simulink library "gnss_sdr_tcp_connector_tracking_lib"  (Simulink 7.6)
settings: Solver=VariableStepDiscrete  StartTime=0.0  StopTime=10.0  RelTol=1e-3
undefined symbols (not defined in the file or in its folder): B_DLL, B_PLL, f0, magnitude, SFunSlope, T, Tc, Ti
libraries: simulink x518, instrumentlib x2, dspindex x1
(part 1 of 4)
settings Model: Creator=David Pubill  LastModifiedBy=gnss

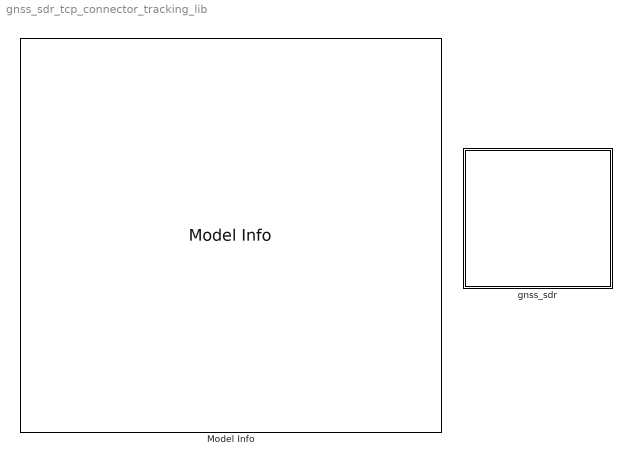
== system gnss_sdr_tcp_connector_tracking_lib ==
  Model Info : simulink/Model-Wide Utilities/Model Info  SystemSampleTime=-1  InitialBlockCM=None  BlockCM=None  Frame=on  DisplayStringWithTags=|  HorizontalTextAlignment=Left  LeftAlignmentValue=0.02  SourceBlockDiagram=gnss_sdr_tcp_connector_tracking_lib  TagMaxNumber=20
      | /*! 
      |   * \file gnss_sdr_tcp_connector_tracking_lib.mdl
      |   * \brief  gnss_sdr_tcp_connector_tracking Simulink library model. For 
      |   * further information, please check  the README_gnss_sdr_tcp_connector_tracking.txt
      |   * file or the README_gnss_sdr_tcp_connector_parallel_tracking.txt
      |   * file for parallel computing execution.
      |   *
      |   * \author David Pubill, 2012. dpubill(at)cttc.es
      |   * -------------------------------------------------------------------------
      |   *
      |   * Copyright (C) 2010-2012  (see AUTHORS file for a list of contributors)
      |   *
      |   * GNSS-SDR is a software defined Global Navigation
      |   *          Satellite Systems receiver
      |   *
      |   * This file is part of GNSS-SDR.
      |   *
      |   * GNSS-SDR is free software: you can redistribute it and/or modify
      |   * it under the terms of the GNU General Public License as published by
      |   * the Free Software Foundation, either version 3 of the License, or
      |   * at your option) any later version.
      |   *
      |   * GNSS-SDR is distributed in the hope that it will be useful,
      |   * but WITHOUT ANY WARRANTY; without even the implied warranty of
      |   * MERCHANTABILITY or FITNESS FOR A PARTICULAR PURPOSE.  See the
      |   * GNU General Public License for more details.
      |   *
      |   * You should have received a copy of the GNU General Public License
      |   * along with GNSS-SDR. If not, see <http://www.gnu.org/licenses/>.
      |   *
      |   * -------------------------------------------------------------------------
      |   */
  gnss_sdr : Subsystem

== system gnss_sdr_tcp_connector_tracking_lib/gnss_sdr ==
  gnss_sdr_tcp_connector_tracking : Subsystem  AncestorBlock=simulink/User-Defined Functions/gnss_sdr/gnss_sdr_tcp_connector_tracking
  gnss_sdr_tcp_connector_tracking_rx : Subsystem
  gnss_sdr_tcp_connector_tracking_tx : Subsystem  AncestorBlock=simulink/User-Defined Functions/gnss_sdr/gnss_sdr_tcp_connector_tracking_tx

== system gnss_sdr_tcp_connector_tracking_lib/gnss_sdr/gnss_sdr_tcp_connector_tracking ==
  control_id : Inport
  d_E_I : Inport  Port=2
  d_E_Q : Inport  Port=3
  d_L_I : Inport  Port=4
  d_L_Q : Inport  Port=5
  d_P_I : Inport  Port=6
  d_P_Q : Inport  Port=7
  d_acq_carrier_doppler_[Hz] : Inport  Port=8
  enable_tracking : Inport  Port=9
  Abs : Abs
  Abs1 : Abs
  Abs2 : Abs
  Carrier Tracking  (PLL) : Subsystem
  Code Tracking (DLL) : Subsystem
  Data Type  Conversion1 : DataTypeConversion  OutDataTypeStr=single  SaturateOnIntegerOverflow=on  RndMeth=Zero
  Data Type  Conversion2 : DataTypeConversion  OutDataTypeStr=double  SaturateOnIntegerOverflow=on  RndMeth=Zero
  Data Type  Conversion3 : DataTypeConversion  OutDataTypeStr=single  SaturateOnIntegerOverflow=on  RndMeth=Zero
  Data Type  Conversion4 : DataTypeConversion  OutDataTypeStr=single  SaturateOnIntegerOverflow=on  RndMeth=Zero
  Data Type  Conversion5 : DataTypeConversion  OutDataTypeStr=double  SaturateOnIntegerOverflow=on  RndMeth=Zero
  Data Type  Conversion6 : DataTypeConversion  OutDataTypeStr=double  SaturateOnIntegerOverflow=on  RndMeth=Zero
  Mux : Mux  Inputs=3
  Real-Imag to Complex : RealImagToComplex
  Real-Imag to Complex1 : RealImagToComplex
  Real-Imag to Complex2 : RealImagToComplex
  "[rad/s] to [Hz]" : Gain  Gain=1/(2*pi)
  control_id_ : Outport
  code_error_[s] : Outport  Port=2
  carrier_error : Outport  Port=3
  carrier_doppler_[Hz] : Outport  Port=4
  EPL Scope : Outport  Port=5
  wires:
  Carrier Tracking  (PLL)/2(carrier_doppler) -> Code Tracking (DLL)/4(carrier_aid), "[rad/s] to [Hz]"/1
  Code Tracking (DLL)/1(code_error [s]) -> Data Type  Conversion1/1
  Real-Imag to Complex/1 -> Data Type  Conversion2/1
  Carrier Tracking  (PLL)/1(carrier_error) -> Data Type  Conversion4/1
  Real-Imag to Complex1/1 -> Data Type  Conversion5/1
  Real-Imag to Complex2/1 -> Data Type  Conversion6/1
  d_E_I/1 -> Real-Imag to Complex/1
  d_E_Q/1 -> Real-Imag to Complex/2
  Data Type  Conversion1/1 -> code_error_[s]/1
  Data Type  Conversion4/1 -> carrier_error/1
  control_id/1 -> control_id_/1
  d_L_I/1 -> Real-Imag to Complex1/1
  d_L_Q/1 -> Real-Imag to Complex1/2
  d_P_I/1 -> Real-Imag to Complex2/1
  d_P_Q/1 -> Real-Imag to Complex2/2
  Data Type  Conversion2/1 -> Code Tracking (DLL)/1(E), Abs2/1
  Data Type  Conversion5/1 -> Code Tracking (DLL)/3(L), Abs/1
  Data Type  Conversion6/1 -> Carrier Tracking  (PLL)/1(P), Code Tracking (DLL)/2(P), Abs1/1
  d_acq_carrier_doppler_[Hz]/1 -> Carrier Tracking  (PLL)/2(d_acq_carrier_doppler_[Hz])
  "[rad/s] to [Hz]"/1 -> Data Type  Conversion3/1
  Data Type  Conversion3/1 -> carrier_doppler_[Hz]/1
  enable_tracking/1 -> Carrier Tracking  (PLL)/3(enable_tracking)
  Abs/1 -> Mux/3
  Abs1/1 -> Mux/2
  Abs2/1 -> Mux/1
  Mux/1 -> EPL Scope/1

== system gnss_sdr_tcp_connector_tracking_lib/gnss_sdr/gnss_sdr_tcp_connector_tracking_rx ==
  Multiport Selector : dspindex/Multiport Selector  rowsOrCols=Rows  idxCellArray={1,2,3,4,5,6,7,8,9,10,11,12,13,14,15,16,17,18,19,20,21,22,23,24,25,26,27,28,29,30,31,32,33,34,35,36}  idxErrMode=Clip Index
  RX : instrumentlib/TCP//IP Receive  DialogController=instrumentcreatedialog  DialogControllerArgs=DataTag4  Host=84.88.61.86  Port=2070  DataSize=36  EnableBlockingMode=on  Timeout=5  SampleTime=-1  DataType=uint8  ByteOrder=BigEndian
  Subsystem : Subsystem
  Subsystem1 : Subsystem
  Subsystem2 : Subsystem
  Subsystem3 : Subsystem
  Subsystem4 : Subsystem
  Subsystem5 : Subsystem
  Subsystem6 : Subsystem
  Subsystem7 : Subsystem
  Subsystem8 : Subsystem
  control_id : Outport
  d_E_I : Outport  Port=2
  d_E_Q : Outport  Port=3
  d_L_I : Outport  Port=4
  d_L_Q : Outport  Port=5
  d_P_I : Outport  Port=6
  d_P_Q : Outport  Port=7
  d_acq_carrier_doppler_hz : Outport  Port=8
  enable_tracking : Outport  Port=9
  wires:
  RX/1 -> Multiport Selector/1
  Multiport Selector/1 -> Subsystem8/1(In1)
  Multiport Selector/2 -> Subsystem8/2(In2)
  Multiport Selector/3 -> Subsystem8/3(In3)
  Multiport Selector/4 -> Subsystem8/4(In4)
  Multiport Selector/5 -> Subsystem/1(In1)
  Multiport Selector/6 -> Subsystem/2(In2)
  Multiport Selector/7 -> Subsystem/3(In3)
  Multiport Selector/8 -> Subsystem/4(In4)
  Multiport Selector/9 -> Subsystem1/1(In1)
  Multiport Selector/10 -> Subsystem1/2(In2)
  Multiport Selector/11 -> Subsystem1/3(In3)
  Multiport Selector/12 -> Subsystem1/4(In4)
  Multiport Selector/13 -> Subsystem2/1(In1)
  Multiport Selector/14 -> Subsystem2/2(In2)
  Multiport Selector/15 -> Subsystem2/3(In3)
  Multiport Selector/16 -> Subsystem2/4(In4)
  Multiport Selector/17 -> Subsystem3/1(In1)
  Multiport Selector/18 -> Subsystem3/2(In2)
  Multiport Selector/19 -> Subsystem3/3(In3)
  Multiport Selector/20 -> Subsystem3/4(In4)
  Multiport Selector/21 -> Subsystem4/1(In1)
  Multiport Selector/22 -> Subsystem4/2(In2)
  Multiport Selector/23 -> Subsystem4/3(In3)
  Multiport Selector/24 -> Subsystem4/4(In4)
  Multiport Selector/25 -> Subsystem5/1(In1)
  Multiport Selector/26 -> Subsystem5/2(In2)
  Multiport Selector/27 -> Subsystem5/3(In3)
  Multiport Selector/28 -> Subsystem5/4(In4)
  Subsystem4/1(d_P_I) -> d_P_I/1
  Subsystem3/1(d_L_Q) -> d_L_Q/1
  Subsystem2/1(d_L_I) -> d_L_I/1
  Subsystem1/1(d_E_Q) -> d_E_Q/1
  Subsystem/1(d_E_I) -> d_E_I/1
  Subsystem8/1(control_id) -> control_id/1
  Subsystem5/1(d_P_Q) -> d_P_Q/1
  Multiport Selector/29 -> Subsystem6/1(In1)
  Multiport Selector/30 -> Subsystem6/2(In2)
  Multiport Selector/31 -> Subsystem6/3(In3)
  Multiport Selector/32 -> Subsystem6/4(In4)
  Subsystem6/1(d_acq_carrier_doppler_hz) -> d_acq_carrier_doppler_hz/1
  Subsystem7/1(enable_tracking) -> enable_tracking/1
  Multiport Selector/33 -> Subsystem7/1(In1)
  Multiport Selector/34 -> Subsystem7/2(In2)
  Multiport Selector/35 -> Subsystem7/3(In3)
  Multiport Selector/36 -> Subsystem7/4(In4)

== system gnss_sdr_tcp_connector_tracking_lib/gnss_sdr/gnss_sdr_tcp_connector_tracking_tx ==
  control_id : Inport
  code_error : Inport  Port=2
  carr_error : Inport  Port=3
  carrier_doppler_hz : Inport  Port=4
  Display : Display
  TX : instrumentlib/TCP//IP Send  DialogController=instrumentcreatedialog  DialogControllerArgs=DataTag5  Host=84.88.61.86  Port=2070  EnableBlockingMode=on  Timeout=10  ByteOrder=LittleEndian
  Vector Concatenate1 : Concatenate  NumInputs=4  Mode=Vector
  wires:
  carr_error/1 -> Vector Concatenate1/3
  code_error/1 -> Vector Concatenate1/2
  control_id/1 -> Vector Concatenate1/1
  Vector Concatenate1/1 -> TX/1, Display/1
  carrier_doppler_hz/1 -> Vector Concatenate1/4

== system gnss_sdr_tcp_connector_tracking_lib/gnss_sdr/gnss_sdr_tcp_connector_tracking/Carrier Tracking  (PLL) ==
  P : Inport
  d_acq_carrier_doppler_[Hz] : Inport  Port=2
  enable_tracking : Inport  Port=3
  Data Type  Conversion2 : DataTypeConversion  OutDataTypeStr=double  SaturateOnIntegerOverflow=on  RndMeth=Zero
  Delay : simulink/Discrete/Integer Delay  NumDelays=1  InputProcessing=Inherited  vinit=0.0  samptime=Ti
  Error Accumulator : Subsystem
  First-Order Low-Pass Filter : Subsystem
  PLL Costas loop two  quadrant arctan discriminator : Subsystem  AncestorBlock=|
      | gnss_sdr_tcp_connector_tracking_lib/gnss_sdr/gnss_sdr_tcp_connector_tracking/Carrier Tracking 
      | (PLL)/atan2(Q,I)1/PLL Costas loop two quadrant arctan discriminator
  Sum : Sum  Inputs=|++
  Sum2 : Sum  Inputs=++|
  "[Hz] to [rad/Ti]" : Gain  Gain=2*pi*Ti  SaturateOnIntegerOverflow=on  OutDataTypeStr=Inherit: Same as input  ParamDataTypeStr=Inherit: Same as input
  "[rad/Ti] to [rad/s]" : Gain  Gain=1/Ti
  carrier_error : Outport
  carrier_doppler : Outport  Port=2
  wires:
  Sum/1 -> Error Accumulator/1(e)
  Error Accumulator/1(sum(e)) -> carrier_error/1
  P/1 -> PLL Costas loop two  quadrant arctan discriminator/1(In)
  "[rad/Ti] to [rad/s]"/1 -> carrier_doppler/1
  Delay/1 -> Sum/2
  Sum2/1 -> "[rad/Ti] to [rad/s]"/1
  d_acq_carrier_doppler_[Hz]/1 -> Data Type  Conversion2/1
  Data Type  Conversion2/1 -> "[Hz] to [rad/Ti]"/1
  enable_tracking/1 -> Error Accumulator/2(enable_tracking)
  "[Hz] to [rad/Ti]"/1 -> Delay/1, Sum2/2
  First-Order Low-Pass Filter/1(Out) -> Sum/1, Sum2/1
  PLL Costas loop two  quadrant arctan discriminator/1(Out) -> First-Order Low-Pass Filter/1(In)

== system gnss_sdr_tcp_connector_tracking_lib/gnss_sdr/gnss_sdr_tcp_connector_tracking/Code Tracking (DLL) ==
  E : Inport
  P : Inport  Port=2
  L : Inport  Port=3
  carrier_aid : Inport  Port=4
  Delay : simulink/Discrete/Integer Delay  NumDelays=1  InputProcessing=Inherited  vinit=0.0  samptime=Ti
  Early-Late Power : Subsystem
  Gain : Gain  Gain=-1
  Normalization : Subsystem
  Sum : Sum  Inputs=|++
  Terminator : Terminator
  Zero Order Low-Pass Filter : Subsystem
  "[chip] to [s]" : Gain  Gain=Tc  SaturateOnIntegerOverflow=on  OutDataTypeStr=Inherit: Same as input  ParamDataTypeStr=Inherit: Same as input
  "[rad/s] to [s/Ti]" : Gain  Gain=-Ti/(2*pi*f0)
  code_error [s] : Outport
  wires:
  Gain/1 -> Zero Order Low-Pass Filter/1(in)
  L/1 -> Normalization/3(L)
  P/1 -> Normalization/2(P)
  E/1 -> Normalization/1(E)
  "[chip] to [s]"/1 -> Gain/1
  Early-Late Power/1(Tau) -> "[chip] to [s]"/1
  "[rad/s] to [s/Ti]"/1 -> Delay/1
  carrier_aid/1 -> "[rad/s] to [s/Ti]"/1
  Sum/1 -> code_error [s]/1
  Delay/1 -> Sum/2
  Normalization/3(L') -> Early-Late Power/2(L)
  Normalization/1(E') -> Early-Late Power/1(E)
  Normalization/2(P') -> Terminator/1
  Zero Order Low-Pass Filter/1(out) -> Sum/1

== system gnss_sdr_tcp_connector_tracking_lib/gnss_sdr/gnss_sdr_tcp_connector_tracking_rx/Subsystem ==
  In1 : Inport
  In2 : Inport  Port=2
  In3 : Inport  Port=3
  In4 : Inport  Port=4
  Data Type  Conversion{1..5} (5 alike) : DataTypeConversion  OutDataTypeStr=single  SaturateOnIntegerOverflow=on  RndMeth=Zero
  hex2float : Subsystem
  d_E_I : Outport  OutputWhenDisabled=reset  InitialOutput=0
  wires:
  Data Type  Conversion5/1 -> d_E_I/1
  hex2float/1(Out1) -> Data Type  Conversion5/1
  Data Type  Conversion4/1 -> hex2float/1(In1)
  Data Type  Conversion1/1 -> hex2float/2(In2)
  Data Type  Conversion2/1 -> hex2float/3(In3)
  Data Type  Conversion3/1 -> hex2float/4(In4)
  In4/1 -> Data Type  Conversion4/1
  In3/1 -> Data Type  Conversion1/1
  In2/1 -> Data Type  Conversion2/1
  In1/1 -> Data Type  Conversion3/1

== system gnss_sdr_tcp_connector_tracking_lib/gnss_sdr/gnss_sdr_tcp_connector_tracking_rx/Subsystem1 ==
  In1 : Inport
  In2 : Inport  Port=2
  In3 : Inport  Port=3
  In4 : Inport  Port=4
  Data Type  Conversion{1..5} (5 alike) : DataTypeConversion  OutDataTypeStr=single  SaturateOnIntegerOverflow=on  RndMeth=Zero
  hex2float : Subsystem
  d_E_Q : Outport  OutputWhenDisabled=reset  InitialOutput=0
  wires:
  In1/1 -> Data Type  Conversion3/1
  In2/1 -> Data Type  Conversion2/1
  In3/1 -> Data Type  Conversion1/1
  In4/1 -> Data Type  Conversion4/1
  Data Type  Conversion3/1 -> hex2float/4(In4)
  Data Type  Conversion2/1 -> hex2float/3(In3)
  Data Type  Conversion1/1 -> hex2float/2(In2)
  Data Type  Conversion4/1 -> hex2float/1(In1)
  hex2float/1(Out1) -> Data Type  Conversion5/1
  Data Type  Conversion5/1 -> d_E_Q/1

== system gnss_sdr_tcp_connector_tracking_lib/gnss_sdr/gnss_sdr_tcp_connector_tracking_rx/Subsystem2 ==
  In1 : Inport
  In2 : Inport  Port=2
  In3 : Inport  Port=3
  In4 : Inport  Port=4
  Data Type  Conversion{1..5} (5 alike) : DataTypeConversion  OutDataTypeStr=single  SaturateOnIntegerOverflow=on  RndMeth=Zero
  hex2float : Subsystem
  d_L_I : Outport  OutputWhenDisabled=reset  InitialOutput=0
  wires:
  Data Type  Conversion5/1 -> d_L_I/1
  hex2float/1(Out1) -> Data Type  Conversion5/1
  Data Type  Conversion4/1 -> hex2float/1(In1)
  Data Type  Conversion1/1 -> hex2float/2(In2)
  Data Type  Conversion2/1 -> hex2float/3(In3)
  Data Type  Conversion3/1 -> hex2float/4(In4)
  In4/1 -> Data Type  Conversion4/1
  In3/1 -> Data Type  Conversion1/1
  In2/1 -> Data Type  Conversion2/1
  In1/1 -> Data Type  Conversion3/1

== system gnss_sdr_tcp_connector_tracking_lib/gnss_sdr/gnss_sdr_tcp_connector_tracking_rx/Subsystem3 ==
  In1 : Inport
  In2 : Inport  Port=2
  In3 : Inport  Port=3
  In4 : Inport  Port=4
  Data Type  Conversion{1..5} (5 alike) : DataTypeConversion  OutDataTypeStr=single  SaturateOnIntegerOverflow=on  RndMeth=Zero
  hex2float : Subsystem
  d_L_Q : Outport  OutputWhenDisabled=reset  InitialOutput=0
  wires:
  In1/1 -> Data Type  Conversion3/1
  In2/1 -> Data Type  Conversion2/1
  In3/1 -> Data Type  Conversion1/1
  In4/1 -> Data Type  Conversion4/1
  Data Type  Conversion3/1 -> hex2float/4(In4)
  Data Type  Conversion2/1 -> hex2float/3(In3)
  Data Type  Conversion1/1 -> hex2float/2(In2)
  Data Type  Conversion4/1 -> hex2float/1(In1)
  hex2float/1(Out1) -> Data Type  Conversion5/1
  Data Type  Conversion5/1 -> d_L_Q/1

== system gnss_sdr_tcp_connector_tracking_lib/gnss_sdr/gnss_sdr_tcp_connector_tracking_rx/Subsystem4 ==
  In1 : Inport
  In2 : Inport  Port=2
  In3 : Inport  Port=3
  In4 : Inport  Port=4
  Data Type  Conversion{1..5} (5 alike) : DataTypeConversion  OutDataTypeStr=single  SaturateOnIntegerOverflow=on  RndMeth=Zero
  hex2float : Subsystem
  d_P_I : Outport  OutputWhenDisabled=reset  InitialOutput=0
  wires:
  In1/1 -> Data Type  Conversion3/1
  In2/1 -> Data Type  Conversion2/1
  In3/1 -> Data Type  Conversion1/1
  In4/1 -> Data Type  Conversion4/1
  Data Type  Conversion3/1 -> hex2float/4(In4)
  Data Type  Conversion2/1 -> hex2float/3(In3)
  Data Type  Conversion1/1 -> hex2float/2(In2)
  Data Type  Conversion4/1 -> hex2float/1(In1)
  hex2float/1(Out1) -> Data Type  Conversion5/1
  Data Type  Conversion5/1 -> d_P_I/1

== system gnss_sdr_tcp_connector_tracking_lib/gnss_sdr/gnss_sdr_tcp_connector_tracking_rx/Subsystem5 ==
  In1 : Inport
  In2 : Inport  Port=2
  In3 : Inport  Port=3
  In4 : Inport  Port=4
  Data Type  Conversion{1..5} (5 alike) : DataTypeConversion  OutDataTypeStr=single  SaturateOnIntegerOverflow=on  RndMeth=Zero
  hex2float : Subsystem
  d_P_Q : Outport  OutputWhenDisabled=reset  InitialOutput=0
  wires:
  Data Type  Conversion5/1 -> d_P_Q/1
  hex2float/1(Out1) -> Data Type  Conversion5/1
  Data Type  Conversion4/1 -> hex2float/1(In1)
  Data Type  Conversion1/1 -> hex2float/2(In2)
  Data Type  Conversion2/1 -> hex2float/3(In3)
  Data Type  Conversion3/1 -> hex2float/4(In4)
  In4/1 -> Data Type  Conversion4/1
  In3/1 -> Data Type  Conversion1/1
  In2/1 -> Data Type  Conversion2/1
  In1/1 -> Data Type  Conversion3/1

== system gnss_sdr_tcp_connector_tracking_lib/gnss_sdr/gnss_sdr_tcp_connector_tracking_rx/Subsystem6 ==
  In1 : Inport
  In2 : Inport  Port=2
  In3 : Inport  Port=3
  In4 : Inport  Port=4
  Data Type  Conversion{1..5} (5 alike) : DataTypeConversion  OutDataTypeStr=single  SaturateOnIntegerOverflow=on  RndMeth=Zero
  hex2float : Subsystem
  d_acq_carrier_doppler_hz : Outport  OutputWhenDisabled=reset  InitialOutput=0
  wires:
  In1/1 -> Data Type  Conversion3/1
  In2/1 -> Data Type  Conversion2/1
  In3/1 -> Data Type  Conversion1/1
  In4/1 -> Data Type  Conversion4/1
  Data Type  Conversion3/1 -> hex2float/4(In4)
  Data Type  Conversion2/1 -> hex2float/3(In3)
  Data Type  Conversion1/1 -> hex2float/2(In2)
  Data Type  Conversion4/1 -> hex2float/1(In1)
  hex2float/1(Out1) -> Data Type  Conversion5/1
  Data Type  Conversion5/1 -> d_acq_carrier_doppler_hz/1

== system gnss_sdr_tcp_connector_tracking_lib/gnss_sdr/gnss_sdr_tcp_connector_tracking_rx/Subsystem7 ==
  In1 : Inport
  In2 : Inport  Port=2
  In3 : Inport  Port=3
  In4 : Inport  Port=4
  Data Type  Conversion{1..5} (5 alike) : DataTypeConversion  OutDataTypeStr=single  SaturateOnIntegerOverflow=on  RndMeth=Zero
  hex2float : Subsystem
  enable_tracking : Outport  OutputWhenDisabled=reset  InitialOutput=0
  wires:
  Data Type  Conversion5/1 -> enable_tracking/1
  hex2float/1(Out1) -> Data Type  Conversion5/1
  Data Type  Conversion4/1 -> hex2float/1(In1)
  Data Type  Conversion1/1 -> hex2float/2(In2)
  Data Type  Conversion2/1 -> hex2float/3(In3)
  Data Type  Conversion3/1 -> hex2float/4(In4)
  In4/1 -> Data Type  Conversion4/1
  In3/1 -> Data Type  Conversion1/1
  In2/1 -> Data Type  Conversion2/1
  In1/1 -> Data Type  Conversion3/1

== system gnss_sdr_tcp_connector_tracking_lib/gnss_sdr/gnss_sdr_tcp_connector_tracking_rx/Subsystem8 ==
  In1 : Inport
  In2 : Inport  Port=2
  In3 : Inport  Port=3
  In4 : Inport  Port=4
  Data Type  Conversion{1..5} (5 alike) : DataTypeConversion  OutDataTypeStr=single  SaturateOnIntegerOverflow=on  RndMeth=Zero
  hex2float : Subsystem
  control_id : Outport  OutputWhenDisabled=reset  InitialOutput=0
  wires:
  Data Type  Conversion5/1 -> control_id/1
  hex2float/1(Out1) -> Data Type  Conversion5/1
  Data Type  Conversion4/1 -> hex2float/1(In1)
  Data Type  Conversion1/1 -> hex2float/2(In2)
  Data Type  Conversion2/1 -> hex2float/3(In3)
  Data Type  Conversion3/1 -> hex2float/4(In4)
  In4/1 -> Data Type  Conversion4/1
  In3/1 -> Data Type  Conversion1/1
  In2/1 -> Data Type  Conversion2/1
  In1/1 -> Data Type  Conversion3/1

== system gnss_sdr_tcp_connector_tracking_lib/gnss_sdr/gnss_sdr_tcp_connector_tracking/Carrier Tracking  (PLL)/Error Accumulator ==
  e : Inport
  enable_tracking : Inport  Port=2
  Constant : Constant  Value=0  SampleTime=-1
  Sum2 : Sum  Inputs=|++  SaturateOnIntegerOverflow=on
  Switch : Switch  Threshold=1
  Unit Delay : UnitDelay  SampleTime=-1
  sum(e) : Outport
  wires:
  e/1 -> Sum2/1
  Unit Delay/1 -> Sum2/2
  Sum2/1 -> Switch/1
  Switch/1 -> sum(e)/1, Unit Delay/1
  enable_tracking/1 -> Switch/2
  Constant/1 -> Switch/3

== system gnss_sdr_tcp_connector_tracking_lib/gnss_sdr/gnss_sdr_tcp_connector_tracking/Carrier Tracking  (PLL)/First-Order Low-Pass Filter ==
  In : Inport
  B : Constant  Value=B_PLL  SampleTime=T
  Product : Product  RndMeth=Zero
  Product1 : Product  RndMeth=Zero
  Sum : Sum  Inputs=|++  SampleTime=T  SaturateOnIntegerOverflow=on
  Sum1 : Sum  Inputs=|++  SaturateOnIntegerOverflow=on
  Unit Delay : UnitDelay  SampleTime=T
  gamma : Gain  Gain=(16*(0.707)^2*T) / (1 + 4*(0.707)^2);
  rho : Gain  Gain=(4*T) / (1 + 4*(0.707)^2)
  Out : Outport
  wires:
  rho/1 -> Product/2
  gamma/1 -> Product1/2
  B/1 -> rho/1, gamma/1
  Product/1 -> Sum1/1
  Product1/1 -> Product/1, Sum/1
  Sum1/1 -> Sum/2, Unit Delay/1
  Unit Delay/1 -> Sum1/2
  In/1 -> Product1/1
  Sum/1 -> Out/1

== system gnss_sdr_tcp_connector_tracking_lib/gnss_sdr/gnss_sdr_tcp_connector_tracking/Carrier Tracking  (PLL)/PLL Costas loop two  quadrant arctan discriminator ==
  In : Inport
  Complex to Real-Imag : ComplexToRealImag
  Divide : Product  Inputs=*/
  Trigonometric Function : Trigonometry  Operator=atan
  Out : Outport
  wires:
  Divide/1 -> Trigonometric Function/1
  Complex to Real-Imag/1 -> Divide/1
  In/1 -> Complex to Real-Imag/1
  Trigonometric Function/1 -> Out/1
  Complex to Real-Imag/2 -> Divide/2

== system gnss_sdr_tcp_connector_tracking_lib/gnss_sdr/gnss_sdr_tcp_connector_tracking/Code Tracking (DLL)/Early-Late Power ==
  E : Inport
  L : Inport  Port=2
  E power : Math  Operator=magnitude^2  SaturateOnIntegerOverflow=on
  L power : Math  Operator=magnitude^2  SaturateOnIntegerOverflow=on
  Sum : Sum  Inputs=+|-  SaturateOnIntegerOverflow=on
  to [chip] : Gain  Gain=1/SFunSlope  SaturateOnIntegerOverflow=on  OutDataTypeStr=Inherit: Same as input  ParamDataTypeStr=Inherit: Same as input
  Tau : Outport
  wires:
  to [chip]/1 -> Tau/1
  Sum/1 -> to [chip]/1
  L power/1 -> Sum/2
  E power/1 -> Sum/1
  E/1 -> E power/1
  L/1 -> L power/1

== system gnss_sdr_tcp_connector_tracking_lib/gnss_sdr/gnss_sdr_tcp_connector_tracking/Code Tracking (DLL)/Normalization ==
  E : Inport
  P : Inport  Port=2
  L : Inport  Port=3
  E Normalisation : Product  Inputs=*/  SaturateOnIntegerOverflow=on  OutDataTypeStr=Inherit: Same as first input
  L Normalisation : Product  Inputs=*/  SaturateOnIntegerOverflow=on  OutDataTypeStr=Inherit: Same as first input
  P Normalisation : Product  Inputs=*/  SaturateOnIntegerOverflow=on  OutDataTypeStr=Inherit: Same as first input
  Power Estimation : Subsystem
  E' : Outport
  P' : Outport  Port=2
  L' : Outport  Port=3
  wires:
  P/1 -> P Normalisation/1, Power Estimation/1(in)
  E/1 -> E Normalisation/1
  E Normalisation/1 -> E'/1
  P Normalisation/1 -> P'/1
  L/1 -> L Normalisation/1
  L Normalisation/1 -> L'/1
  Power Estimation/1(out) -> E Normalisation/2, P Normalisation/2, L Normalisation/2

== system gnss_sdr_tcp_connector_tracking_lib/gnss_sdr/gnss_sdr_tcp_connector_tracking/Code Tracking (DLL)/Zero Order Low-Pass Filter ==
  in : Inport
  B : Constant  Value=B_DLL  SampleTime=T
  Fcn : Fcn  Expr=(4*u*T) / (1 + 2*u*T);
  Product : Product  RndMeth=Zero
  out : Outport
  wires:
  Fcn/1 -> Product/2
  B/1 -> Fcn/1
  Product/1 -> out/1
  in/1 -> Product/1

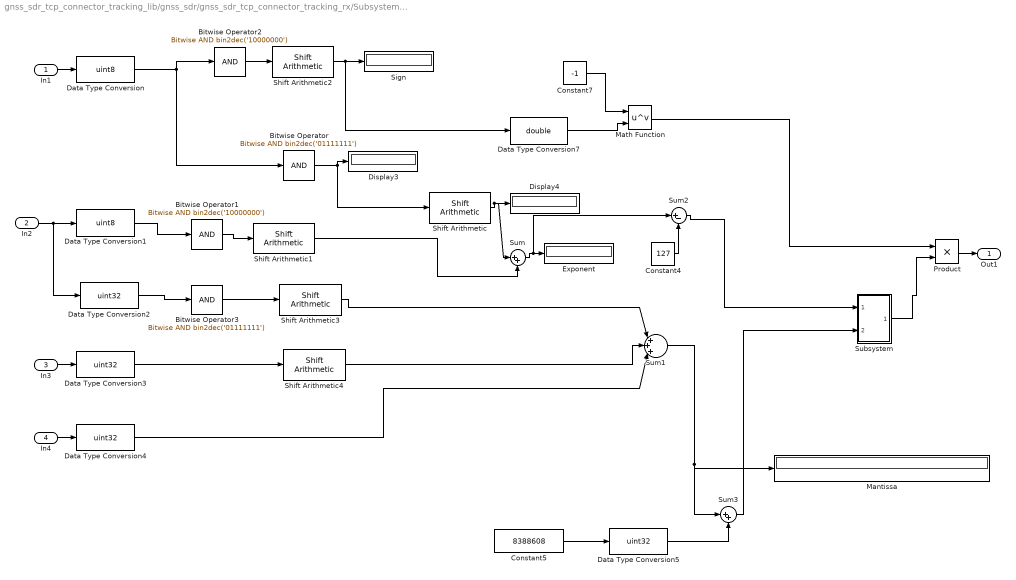
== system gnss_sdr_tcp_connector_tracking_lib/gnss_sdr/gnss_sdr_tcp_connector_tracking_rx/Subsystem/hex2float ==
  In1 : Inport
  In2 : Inport  Port=2
  In3 : Inport  Port=3
  In4 : Inport  Port=4
  Bitwise Operator : simulink/Logic and Bit Operations/Bitwise Operator  logicop=AND  UseBitMask=on  BitMask=bin2dec('01111111')  BitMaskRealWorld=Stored Integer
  Bitwise Operator1 : simulink/Logic and Bit Operations/Bitwise Operator  logicop=AND  UseBitMask=on  BitMask=bin2dec('10000000')  BitMaskRealWorld=Stored Integer
  Bitwise Operator2 : simulink/Logic and Bit Operations/Bitwise Operator  logicop=AND  UseBitMask=on  BitMask=bin2dec('10000000')  BitMaskRealWorld=Stored Integer
  Bitwise Operator3 : simulink/Logic and Bit Operations/Bitwise Operator  logicop=AND  UseBitMask=on  BitMask=bin2dec('01111111')  BitMaskRealWorld=Stored Integer
  Constant4 : Constant  Value=127
  Constant5 : Constant  Value=8388608
  Constant7 : Constant  Value=-1
  Data Type Conversion : DataTypeConversion  OutDataTypeStr=uint8
  Data Type Conversion1 : DataTypeConversion  OutDataTypeStr=uint8
  Data Type Conversion{2..5} (4 alike) : DataTypeConversion  OutDataTypeStr=uint32
  Data Type Conversion7 : DataTypeConversion  OutDataTypeStr=double
  Display3 : Display
      settings: Format=binary (Stored Integer)
  Display4 : Display
      settings: Format=binary (Stored Integer)
  Exponent : Display
      settings: Format=binary (Stored Integer)
  Mantissa : Display
      settings: Format=binary (Stored Integer)
  Math Function : Math  Operator=pow  SaturateOnIntegerOverflow=on
  Product : Product  RndMeth=Zero
  Shift Arithmetic : simulink/Logic and Bit Operations/Shift Arithmetic  SystemSampleTime=-1  nBitShiftRight=-1  nBinPtShiftRight=0
  Shift Arithmetic1 : simulink/Logic and Bit Operations/Shift Arithmetic  SystemSampleTime=-1  nBitShiftRight=7  nBinPtShiftRight=0
  Shift Arithmetic2 : simulink/Logic and Bit Operations/Shift Arithmetic  SystemSampleTime=-1  nBitShiftRight=7  nBinPtShiftRight=0
  Shift Arithmetic3 : simulink/Logic and Bit Operations/Shift Arithmetic  SystemSampleTime=-1  nBitShiftRight=-16  nBinPtShiftRight=0
  Shift Arithmetic4 : simulink/Logic and Bit Operations/Shift Arithmetic  SystemSampleTime=-1  nBitShiftRight=-8  nBinPtShiftRight=0
  Sign : Display
      settings: Format=binary (Stored Integer)
  Subsystem : Subsystem
  Sum : Sum  Inputs=|++
  Sum1 : Sum  Inputs=|+++|
  Sum2 : Sum  Inputs=|+-
  Sum3 : Sum  Inputs=|++
  Out1 : Outport
  wires:
  Bitwise Operator/1 -> Display3/1, Shift Arithmetic/1
  Data Type Conversion/1 -> Bitwise Operator/1, Bitwise Operator2/1
  In2/1 -> Data Type Conversion2/1, Data Type Conversion1/1
  Data Type Conversion1/1 -> Bitwise Operator1/1
  Shift Arithmetic/1 -> Display4/1, Sum/1
  Bitwise Operator1/1 -> Shift Arithmetic1/1
  Shift Arithmetic1/1 -> Sum/2
  Sum/1 -> Exponent/1, Sum2/1
  Bitwise Operator2/1 -> Shift Arithmetic2/1
  Shift Arithmetic2/1 -> Sign/1, Data Type Conversion7/1
  Bitwise Operator3/1 -> Shift Arithmetic3/1
  Data Type Conversion2/1 -> Bitwise Operator3/1
  Shift Arithmetic3/1 -> Sum1/1
  Data Type Conversion3/1 -> Shift Arithmetic4/1
  Shift Arithmetic4/1 -> Sum1/2
  Data Type Conversion4/1 -> Sum1/3
  Sum1/1 -> Mantissa/1, Sum3/1
  Constant4/1 -> Sum2/2
  Sum2/1 -> Subsystem/1(In1)
  Sum3/1 -> Subsystem/2(In2)
  Constant5/1 -> Data Type Conversion5/1
  Data Type Conversion5/1 -> Sum3/2
  Subsystem/1(Out1) -> Product/2
  Constant7/1 -> Math Function/1
  Data Type Conversion7/1 -> Math Function/2
  Math Function/1 -> Product/1
  In1/1 -> Data Type Conversion/1
  Product/1 -> Out1/1
  In3/1 -> Data Type Conversion3/1
  In4/1 -> Data Type Conversion4/1

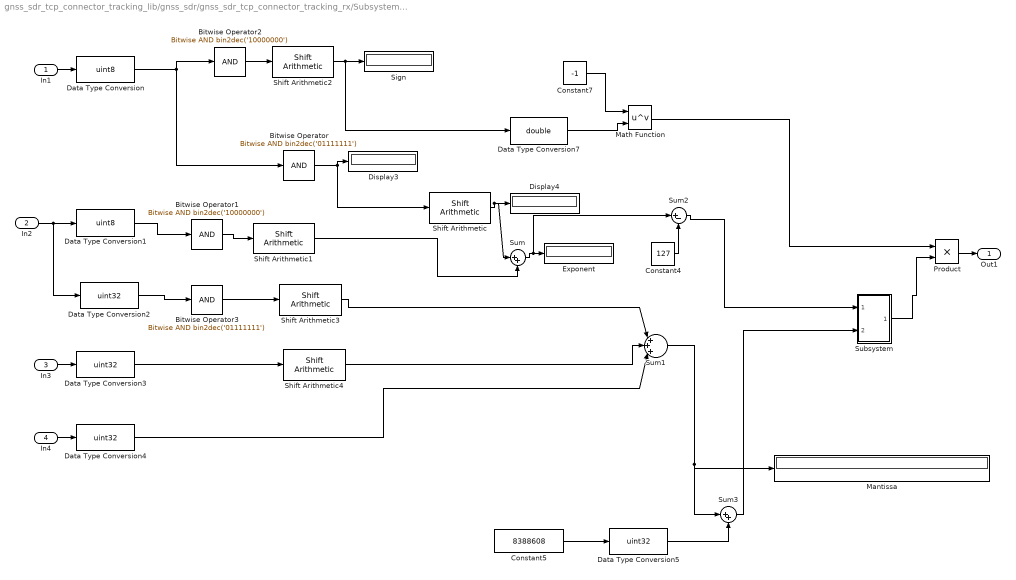
== system gnss_sdr_tcp_connector_tracking_lib/gnss_sdr/gnss_sdr_tcp_connector_tracking_rx/Subsystem1/hex2float ==
  In1 : Inport
  In2 : Inport  Port=2
  In3 : Inport  Port=3
  In4 : Inport  Port=4
  Bitwise Operator : simulink/Logic and Bit Operations/Bitwise Operator  logicop=AND  UseBitMask=on  BitMask=bin2dec('01111111')  BitMaskRealWorld=Stored Integer
  Bitwise Operator1 : simulink/Logic and Bit Operations/Bitwise Operator  logicop=AND  UseBitMask=on  BitMask=bin2dec('10000000')  BitMaskRealWorld=Stored Integer
  Bitwise Operator2 : simulink/Logic and Bit Operations/Bitwise Operator  logicop=AND  UseBitMask=on  BitMask=bin2dec('10000000')  BitMaskRealWorld=Stored Integer
  Bitwise Operator3 : simulink/Logic and Bit Operations/Bitwise Operator  logicop=AND  UseBitMask=on  BitMask=bin2dec('01111111')  BitMaskRealWorld=Stored Integer
  Constant4 : Constant  Value=127
  Constant5 : Constant  Value=8388608
  Constant7 : Constant  Value=-1
  Data Type Conversion : DataTypeConversion  OutDataTypeStr=uint8
  Data Type Conversion1 : DataTypeConversion  OutDataTypeStr=uint8
  Data Type Conversion{2..5} (4 alike) : DataTypeConversion  OutDataTypeStr=uint32
  Data Type Conversion7 : DataTypeConversion  OutDataTypeStr=double
  Display3 : Display
      settings: Format=binary (Stored Integer)
  Display4 : Display
      settings: Format=binary (Stored Integer)
  Exponent : Display
      settings: Format=binary (Stored Integer)
  Mantissa : Display
      settings: Format=binary (Stored Integer)
  Math Function : Math  Operator=pow  SaturateOnIntegerOverflow=on
  Product : Product  RndMeth=Zero
  Shift Arithmetic : simulink/Logic and Bit Operations/Shift Arithmetic  SystemSampleTime=-1  nBitShiftRight=-1  nBinPtShiftRight=0
  Shift Arithmetic1 : simulink/Logic and Bit Operations/Shift Arithmetic  SystemSampleTime=-1  nBitShiftRight=7  nBinPtShiftRight=0
  Shift Arithmetic2 : simulink/Logic and Bit Operations/Shift Arithmetic  SystemSampleTime=-1  nBitShiftRight=7  nBinPtShiftRight=0
  Shift Arithmetic3 : simulink/Logic and Bit Operations/Shift Arithmetic  SystemSampleTime=-1  nBitShiftRight=-16  nBinPtShiftRight=0
  Shift Arithmetic4 : simulink/Logic and Bit Operations/Shift Arithmetic  SystemSampleTime=-1  nBitShiftRight=-8  nBinPtShiftRight=0
  Sign : Display
      settings: Format=binary (Stored Integer)
  Subsystem : Subsystem
  Sum : Sum  Inputs=|++
  Sum1 : Sum  Inputs=|+++|
  Sum2 : Sum  Inputs=|+-
  Sum3 : Sum  Inputs=|++
  Out1 : Outport
  wires:
  In4/1 -> Data Type Conversion4/1
  In3/1 -> Data Type Conversion3/1
  Product/1 -> Out1/1
  In1/1 -> Data Type Conversion/1
  Math Function/1 -> Product/1
  Data Type Conversion7/1 -> Math Function/2
  Constant7/1 -> Math Function/1
  Subsystem/1(Out1) -> Product/2
  Data Type Conversion5/1 -> Sum3/2
  Constant5/1 -> Data Type Conversion5/1
  Sum3/1 -> Subsystem/2(In2)
  Sum2/1 -> Subsystem/1(In1)
  Constant4/1 -> Sum2/2
  Sum1/1 -> Sum3/1, Mantissa/1
  Data Type Conversion4/1 -> Sum1/3
  Shift Arithmetic4/1 -> Sum1/2
  Data Type Conversion3/1 -> Shift Arithmetic4/1
  Shift Arithmetic3/1 -> Sum1/1
  Data Type Conversion2/1 -> Bitwise Operator3/1
  Bitwise Operator3/1 -> Shift Arithmetic3/1
  Shift Arithmetic2/1 -> Data Type Conversion7/1, Sign/1
  Bitwise Operator2/1 -> Shift Arithmetic2/1
  Sum/1 -> Sum2/1, Exponent/1
  Shift Arithmetic1/1 -> Sum/2
  Bitwise Operator1/1 -> Shift Arithmetic1/1
  Shift Arithmetic/1 -> Sum/1, Display4/1
  Data Type Conversion1/1 -> Bitwise Operator1/1
  In2/1 -> Data Type Conversion1/1, Data Type Conversion2/1
  Data Type Conversion/1 -> Bitwise Operator2/1, Bitwise Operator/1
  Bitwise Operator/1 -> Shift Arithmetic/1, Display3/1

== system gnss_sdr_tcp_connector_tracking_lib/gnss_sdr/gnss_sdr_tcp_connector_tracking_rx/Subsystem2/hex2float ==
  In1 : Inport
  In2 : Inport  Port=2
  In3 : Inport  Port=3
  In4 : Inport  Port=4
  Bitwise Operator : simulink/Logic and Bit Operations/Bitwise Operator  logicop=AND  UseBitMask=on  BitMask=bin2dec('01111111')  BitMaskRealWorld=Stored Integer
  Bitwise Operator1 : simulink/Logic and Bit Operations/Bitwise Operator  logicop=AND  UseBitMask=on  BitMask=bin2dec('10000000')  BitMaskRealWorld=Stored Integer
  Bitwise Operator2 : simulink/Logic and Bit Operations/Bitwise Operator  logicop=AND  UseBitMask=on  BitMask=bin2dec('10000000')  BitMaskRealWorld=Stored Integer
  Bitwise Operator3 : simulink/Logic and Bit Operations/Bitwise Operator  logicop=AND  UseBitMask=on  BitMask=bin2dec('01111111')  BitMaskRealWorld=Stored Integer
  Constant4 : Constant  Value=127
  Constant5 : Constant  Value=8388608
  Constant7 : Constant  Value=-1
  Data Type Conversion : DataTypeConversion  OutDataTypeStr=uint8
  Data Type Conversion1 : DataTypeConversion  OutDataTypeStr=uint8
  Data Type Conversion{2..5} (4 alike) : DataTypeConversion  OutDataTypeStr=uint32
  Data Type Conversion7 : DataTypeConversion  OutDataTypeStr=double
  Display3 : Display
      settings: Format=binary (Stored Integer)
  Display4 : Display
      settings: Format=binary (Stored Integer)
  Exponent : Display
      settings: Format=binary (Stored Integer)
  Mantissa : Display
      settings: Format=binary (Stored Integer)
  Math Function : Math  Operator=pow  SaturateOnIntegerOverflow=on
  Product : Product  RndMeth=Zero
  Shift Arithmetic : simulink/Logic and Bit Operations/Shift Arithmetic  SystemSampleTime=-1  nBitShiftRight=-1  nBinPtShiftRight=0
  Shift Arithmetic1 : simulink/Logic and Bit Operations/Shift Arithmetic  SystemSampleTime=-1  nBitShiftRight=7  nBinPtShiftRight=0
  Shift Arithmetic2 : simulink/Logic and Bit Operations/Shift Arithmetic  SystemSampleTime=-1  nBitShiftRight=7  nBinPtShiftRight=0
  Shift Arithmetic3 : simulink/Logic and Bit Operations/Shift Arithmetic  SystemSampleTime=-1  nBitShiftRight=-16  nBinPtShiftRight=0
  Shift Arithmetic4 : simulink/Logic and Bit Operations/Shift Arithmetic  SystemSampleTime=-1  nBitShiftRight=-8  nBinPtShiftRight=0
  Sign : Display
      settings: Format=binary (Stored Integer)
  Subsystem : Subsystem
  Sum : Sum  Inputs=|++
  Sum1 : Sum  Inputs=|+++|
  Sum2 : Sum  Inputs=|+-
  Sum3 : Sum  Inputs=|++
  Out1 : Outport
  wires:
  Bitwise Operator/1 -> Display3/1, Shift Arithmetic/1
  Data Type Conversion/1 -> Bitwise Operator/1, Bitwise Operator2/1
  In2/1 -> Data Type Conversion2/1, Data Type Conversion1/1
  Data Type Conversion1/1 -> Bitwise Operator1/1
  Shift Arithmetic/1 -> Display4/1, Sum/1
  Bitwise Operator1/1 -> Shift Arithmetic1/1
  Shift Arithmetic1/1 -> Sum/2
  Sum/1 -> Exponent/1, Sum2/1
  Bitwise Operator2/1 -> Shift Arithmetic2/1
  Shift Arithmetic2/1 -> Sign/1, Data Type Conversion7/1
  Bitwise Operator3/1 -> Shift Arithmetic3/1
  Data Type Conversion2/1 -> Bitwise Operator3/1
  Shift Arithmetic3/1 -> Sum1/1
  Data Type Conversion3/1 -> Shift Arithmetic4/1
  Shift Arithmetic4/1 -> Sum1/2
  Data Type Conversion4/1 -> Sum1/3
  Sum1/1 -> Mantissa/1, Sum3/1
  Constant4/1 -> Sum2/2
  Sum2/1 -> Subsystem/1(In1)
  Sum3/1 -> Subsystem/2(In2)
  Constant5/1 -> Data Type Conversion5/1
  Data Type Conversion5/1 -> Sum3/2
  Subsystem/1(Out1) -> Product/2
  Constant7/1 -> Math Function/1
  Data Type Conversion7/1 -> Math Function/2
  Math Function/1 -> Product/1
  In1/1 -> Data Type Conversion/1
  Product/1 -> Out1/1
  In3/1 -> Data Type Conversion3/1
  In4/1 -> Data Type Conversion4/1

== system gnss_sdr_tcp_connector_tracking_lib/gnss_sdr/gnss_sdr_tcp_connector_tracking_rx/Subsystem3/hex2float ==
  In1 : Inport
  In2 : Inport  Port=2
  In3 : Inport  Port=3
  In4 : Inport  Port=4
  Bitwise Operator : simulink/Logic and Bit Operations/Bitwise Operator  logicop=AND  UseBitMask=on  BitMask=bin2dec('01111111')  BitMaskRealWorld=Stored Integer
  Bitwise Operator1 : simulink/Logic and Bit Operations/Bitwise Operator  logicop=AND  UseBitMask=on  BitMask=bin2dec('10000000')  BitMaskRealWorld=Stored Integer
  Bitwise Operator2 : simulink/Logic and Bit Operations/Bitwise Operator  logicop=AND  UseBitMask=on  BitMask=bin2dec('10000000')  BitMaskRealWorld=Stored Integer
  Bitwise Operator3 : simulink/Logic and Bit Operations/Bitwise Operator  logicop=AND  UseBitMask=on  BitMask=bin2dec('01111111')  BitMaskRealWorld=Stored Integer
  Constant4 : Constant  Value=127
  Constant5 : Constant  Value=8388608
  Constant7 : Constant  Value=-1
  Data Type Conversion : DataTypeConversion  OutDataTypeStr=uint8
  Data Type Conversion1 : DataTypeConversion  OutDataTypeStr=uint8
  Data Type Conversion{2..5} (4 alike) : DataTypeConversion  OutDataTypeStr=uint32
  Data Type Conversion7 : DataTypeConversion  OutDataTypeStr=double
  Display3 : Display
      settings: Format=binary (Stored Integer)
  Display4 : Display
      settings: Format=binary (Stored Integer)
  Exponent : Display
      settings: Format=binary (Stored Integer)
  Mantissa : Display
      settings: Format=binary (Stored Integer)
  Math Function : Math  Operator=pow  SaturateOnIntegerOverflow=on
  Product : Product  RndMeth=Zero
  Shift Arithmetic : simulink/Logic and Bit Operations/Shift Arithmetic  SystemSampleTime=-1  nBitShiftRight=-1  nBinPtShiftRight=0
  Shift Arithmetic1 : simulink/Logic and Bit Operations/Shift Arithmetic  SystemSampleTime=-1  nBitShiftRight=7  nBinPtShiftRight=0
  Shift Arithmetic2 : simulink/Logic and Bit Operations/Shift Arithmetic  SystemSampleTime=-1  nBitShiftRight=7  nBinPtShiftRight=0
  Shift Arithmetic3 : simulink/Logic and Bit Operations/Shift Arithmetic  SystemSampleTime=-1  nBitShiftRight=-16  nBinPtShiftRight=0
  Shift Arithmetic4 : simulink/Logic and Bit Operations/Shift Arithmetic  SystemSampleTime=-1  nBitShiftRight=-8  nBinPtShiftRight=0
  Sign : Display
      settings: Format=binary (Stored Integer)
  Subsystem : Subsystem
  Sum : Sum  Inputs=|++
  Sum1 : Sum  Inputs=|+++|
  Sum2 : Sum  Inputs=|+-
  Sum3 : Sum  Inputs=|++
  Out1 : Outport
  wires:
  In4/1 -> Data Type Conversion4/1
  In3/1 -> Data Type Conversion3/1
  Product/1 -> Out1/1
  In1/1 -> Data Type Conversion/1
  Math Function/1 -> Product/1
  Data Type Conversion7/1 -> Math Function/2
  Constant7/1 -> Math Function/1
  Subsystem/1(Out1) -> Product/2
  Data Type Conversion5/1 -> Sum3/2
  Constant5/1 -> Data Type Conversion5/1
  Sum3/1 -> Subsystem/2(In2)
  Sum2/1 -> Subsystem/1(In1)
  Constant4/1 -> Sum2/2
  Sum1/1 -> Sum3/1, Mantissa/1
  Data Type Conversion4/1 -> Sum1/3
  Shift Arithmetic4/1 -> Sum1/2
  Data Type Conversion3/1 -> Shift Arithmetic4/1
  Shift Arithmetic3/1 -> Sum1/1
  Data Type Conversion2/1 -> Bitwise Operator3/1
  Bitwise Operator3/1 -> Shift Arithmetic3/1
  Shift Arithmetic2/1 -> Data Type Conversion7/1, Sign/1
  Bitwise Operator2/1 -> Shift Arithmetic2/1
  Sum/1 -> Sum2/1, Exponent/1
  Shift Arithmetic1/1 -> Sum/2
  Bitwise Operator1/1 -> Shift Arithmetic1/1
  Shift Arithmetic/1 -> Sum/1, Display4/1
  Data Type Conversion1/1 -> Bitwise Operator1/1
  In2/1 -> Data Type Conversion1/1, Data Type Conversion2/1
  Data Type Conversion/1 -> Bitwise Operator2/1, Bitwise Operator/1
  Bitwise Operator/1 -> Shift Arithmetic/1, Display3/1

== system gnss_sdr_tcp_connector_tracking_lib/gnss_sdr/gnss_sdr_tcp_connector_tracking_rx/Subsystem4/hex2float ==
  In1 : Inport
  In2 : Inport  Port=2
  In3 : Inport  Port=3
  In4 : Inport  Port=4
  Bitwise Operator : simulink/Logic and Bit Operations/Bitwise Operator  logicop=AND  UseBitMask=on  BitMask=bin2dec('01111111')  BitMaskRealWorld=Stored Integer
  Bitwise Operator1 : simulink/Logic and Bit Operations/Bitwise Operator  logicop=AND  UseBitMask=on  BitMask=bin2dec('10000000')  BitMaskRealWorld=Stored Integer
  Bitwise Operator2 : simulink/Logic and Bit Operations/Bitwise Operator  logicop=AND  UseBitMask=on  BitMask=bin2dec('10000000')  BitMaskRealWorld=Stored Integer
  Bitwise Operator3 : simulink/Logic and Bit Operations/Bitwise Operator  logicop=AND  UseBitMask=on  BitMask=bin2dec('01111111')  BitMaskRealWorld=Stored Integer
  Constant4 : Constant  Value=127
  Constant5 : Constant  Value=8388608
  Constant7 : Constant  Value=-1
  Data Type Conversion : DataTypeConversion  OutDataTypeStr=uint8
  Data Type Conversion1 : DataTypeConversion  OutDataTypeStr=uint8
  Data Type Conversion{2..5} (4 alike) : DataTypeConversion  OutDataTypeStr=uint32
  Data Type Conversion7 : DataTypeConversion  OutDataTypeStr=double
  Display3 : Display
      settings: Format=binary (Stored Integer)
  Display4 : Display
      settings: Format=binary (Stored Integer)
  Exponent : Display
      settings: Format=binary (Stored Integer)
  Mantissa : Display
      settings: Format=binary (Stored Integer)
  Math Function : Math  Operator=pow  SaturateOnIntegerOverflow=on
  Product : Product  RndMeth=Zero
  Shift Arithmetic : simulink/Logic and Bit Operations/Shift Arithmetic  SystemSampleTime=-1  nBitShiftRight=-1  nBinPtShiftRight=0
  Shift Arithmetic1 : simulink/Logic and Bit Operations/Shift Arithmetic  SystemSampleTime=-1  nBitShiftRight=7  nBinPtShiftRight=0
  Shift Arithmetic2 : simulink/Logic and Bit Operations/Shift Arithmetic  SystemSampleTime=-1  nBitShiftRight=7  nBinPtShiftRight=0
  Shift Arithmetic3 : simulink/Logic and Bit Operations/Shift Arithmetic  SystemSampleTime=-1  nBitShiftRight=-16  nBinPtShiftRight=0
  Shift Arithmetic4 : simulink/Logic and Bit Operations/Shift Arithmetic  SystemSampleTime=-1  nBitShiftRight=-8  nBinPtShiftRight=0
  Sign : Display
      settings: Format=binary (Stored Integer)
  Subsystem : Subsystem
  Sum : Sum  Inputs=|++
  Sum1 : Sum  Inputs=|+++|
  Sum2 : Sum  Inputs=|+-
  Sum3 : Sum  Inputs=|++
  Out1 : Outport
  wires:
  In4/1 -> Data Type Conversion4/1
  In3/1 -> Data Type Conversion3/1
  Product/1 -> Out1/1
  In1/1 -> Data Type Conversion/1
  Math Function/1 -> Product/1
  Data Type Conversion7/1 -> Math Function/2
  Constant7/1 -> Math Function/1
  Subsystem/1(Out1) -> Product/2
  Data Type Conversion5/1 -> Sum3/2
  Constant5/1 -> Data Type Conversion5/1
  Sum3/1 -> Subsystem/2(In2)
  Sum2/1 -> Subsystem/1(In1)
  Constant4/1 -> Sum2/2
  Sum1/1 -> Sum3/1, Mantissa/1
  Data Type Conversion4/1 -> Sum1/3
  Shift Arithmetic4/1 -> Sum1/2
  Data Type Conversion3/1 -> Shift Arithmetic4/1
  Shift Arithmetic3/1 -> Sum1/1
  Data Type Conversion2/1 -> Bitwise Operator3/1
  Bitwise Operator3/1 -> Shift Arithmetic3/1
  Shift Arithmetic2/1 -> Data Type Conversion7/1, Sign/1
  Bitwise Operator2/1 -> Shift Arithmetic2/1
  Sum/1 -> Sum2/1, Exponent/1
  Shift Arithmetic1/1 -> Sum/2
  Bitwise Operator1/1 -> Shift Arithmetic1/1
  Shift Arithmetic/1 -> Sum/1, Display4/1
  Data Type Conversion1/1 -> Bitwise Operator1/1
  In2/1 -> Data Type Conversion1/1, Data Type Conversion2/1
  Data Type Conversion/1 -> Bitwise Operator2/1, Bitwise Operator/1
  Bitwise Operator/1 -> Shift Arithmetic/1, Display3/1

== system gnss_sdr_tcp_connector_tracking_lib/gnss_sdr/gnss_sdr_tcp_connector_tracking_rx/Subsystem5/hex2float ==
  In1 : Inport
  In2 : Inport  Port=2
  In3 : Inport  Port=3
  In4 : Inport  Port=4
  Bitwise Operator : simulink/Logic and Bit Operations/Bitwise Operator  logicop=AND  UseBitMask=on  BitMask=bin2dec('01111111')  BitMaskRealWorld=Stored Integer
  Bitwise Operator1 : simulink/Logic and Bit Operations/Bitwise Operator  logicop=AND  UseBitMask=on  BitMask=bin2dec('10000000')  BitMaskRealWorld=Stored Integer
  Bitwise Operator2 : simulink/Logic and Bit Operations/Bitwise Operator  logicop=AND  UseBitMask=on  BitMask=bin2dec('10000000')  BitMaskRealWorld=Stored Integer
  Bitwise Operator3 : simulink/Logic and Bit Operations/Bitwise Operator  logicop=AND  UseBitMask=on  BitMask=bin2dec('01111111')  BitMaskRealWorld=Stored Integer
  Constant4 : Constant  Value=127
  Constant5 : Constant  Value=8388608
  Constant7 : Constant  Value=-1
  Data Type Conversion : DataTypeConversion  OutDataTypeStr=uint8
  Data Type Conversion1 : DataTypeConversion  OutDataTypeStr=uint8
  Data Type Conversion{2..5} (4 alike) : DataTypeConversion  OutDataTypeStr=uint32
  Data Type Conversion7 : DataTypeConversion  OutDataTypeStr=double
  Display3 : Display
      settings: Format=binary (Stored Integer)
  Display4 : Display
      settings: Format=binary (Stored Integer)
  Exponent : Display
      settings: Format=binary (Stored Integer)
  Mantissa : Display
      settings: Format=binary (Stored Integer)
  Math Function : Math  Operator=pow  SaturateOnIntegerOverflow=on
  Product : Product  RndMeth=Zero
  Shift Arithmetic : simulink/Logic and Bit Operations/Shift Arithmetic  SystemSampleTime=-1  nBitShiftRight=-1  nBinPtShiftRight=0
  Shift Arithmetic1 : simulink/Logic and Bit Operations/Shift Arithmetic  SystemSampleTime=-1  nBitShiftRight=7  nBinPtShiftRight=0
  Shift Arithmetic2 : simulink/Logic and Bit Operations/Shift Arithmetic  SystemSampleTime=-1  nBitShiftRight=7  nBinPtShiftRight=0
  Shift Arithmetic3 : simulink/Logic and Bit Operations/Shift Arithmetic  SystemSampleTime=-1  nBitShiftRight=-16  nBinPtShiftRight=0
  Shift Arithmetic4 : simulink/Logic and Bit Operations/Shift Arithmetic  SystemSampleTime=-1  nBitShiftRight=-8  nBinPtShiftRight=0
  Sign : Display
      settings: Format=binary (Stored Integer)
  Subsystem : Subsystem
  Sum : Sum  Inputs=|++
  Sum1 : Sum  Inputs=|+++|
  Sum2 : Sum  Inputs=|+-
  Sum3 : Sum  Inputs=|++
  Out1 : Outport
  wires:
  Bitwise Operator/1 -> Display3/1, Shift Arithmetic/1
  Data Type Conversion/1 -> Bitwise Operator/1, Bitwise Operator2/1
  In2/1 -> Data Type Conversion2/1, Data Type Conversion1/1
  Data Type Conversion1/1 -> Bitwise Operator1/1
  Shift Arithmetic/1 -> Display4/1, Sum/1
  Bitwise Operator1/1 -> Shift Arithmetic1/1
  Shift Arithmetic1/1 -> Sum/2
  Sum/1 -> Exponent/1, Sum2/1
  Bitwise Operator2/1 -> Shift Arithmetic2/1
  Shift Arithmetic2/1 -> Sign/1, Data Type Conversion7/1
  Bitwise Operator3/1 -> Shift Arithmetic3/1
  Data Type Conversion2/1 -> Bitwise Operator3/1
  Shift Arithmetic3/1 -> Sum1/1
  Data Type Conversion3/1 -> Shift Arithmetic4/1
  Shift Arithmetic4/1 -> Sum1/2
  Data Type Conversion4/1 -> Sum1/3
  Sum1/1 -> Mantissa/1, Sum3/1
  Constant4/1 -> Sum2/2
  Sum2/1 -> Subsystem/1(In1)
  Sum3/1 -> Subsystem/2(In2)
  Constant5/1 -> Data Type Conversion5/1
  Data Type Conversion5/1 -> Sum3/2
  Subsystem/1(Out1) -> Product/2
  Constant7/1 -> Math Function/1
  Data Type Conversion7/1 -> Math Function/2
  Math Function/1 -> Product/1
  In1/1 -> Data Type Conversion/1
  Product/1 -> Out1/1
  In3/1 -> Data Type Conversion3/1
  In4/1 -> Data Type Conversion4/1

== system gnss_sdr_tcp_connector_tracking_lib/gnss_sdr/gnss_sdr_tcp_connector_tracking_rx/Subsystem6/hex2float ==
  In1 : Inport
  In2 : Inport  Port=2
  In3 : Inport  Port=3
  In4 : Inport  Port=4
  Bitwise Operator : simulink/Logic and Bit Operations/Bitwise Operator  logicop=AND  UseBitMask=on  BitMask=bin2dec('01111111')  BitMaskRealWorld=Stored Integer
  Bitwise Operator1 : simulink/Logic and Bit Operations/Bitwise Operator  logicop=AND  UseBitMask=on  BitMask=bin2dec('10000000')  BitMaskRealWorld=Stored Integer
  Bitwise Operator2 : simulink/Logic and Bit Operations/Bitwise Operator  logicop=AND  UseBitMask=on  BitMask=bin2dec('10000000')  BitMaskRealWorld=Stored Integer
  Bitwise Operator3 : simulink/Logic and Bit Operations/Bitwise Operator  logicop=AND  UseBitMask=on  BitMask=bin2dec('01111111')  BitMaskRealWorld=Stored Integer
  Constant4 : Constant  Value=127
  Constant5 : Constant  Value=8388608
  Constant7 : Constant  Value=-1
  Data Type Conversion : DataTypeConversion  OutDataTypeStr=uint8
  Data Type Conversion1 : DataTypeConversion  OutDataTypeStr=uint8
  Data Type Conversion{2..5} (4 alike) : DataTypeConversion  OutDataTypeStr=uint32
  Data Type Conversion7 : DataTypeConversion  OutDataTypeStr=double
  Display3 : Display
      settings: Format=binary (Stored Integer)
  Display4 : Display
      settings: Format=binary (Stored Integer)
  Exponent : Display
      settings: Format=binary (Stored Integer)
  Mantissa : Display
      settings: Format=binary (Stored Integer)
  Math Function : Math  Operator=pow  SaturateOnIntegerOverflow=on
  Product : Product  RndMeth=Zero
  Shift Arithmetic : simulink/Logic and Bit Operations/Shift Arithmetic  SystemSampleTime=-1  nBitShiftRight=-1  nBinPtShiftRight=0
  Shift Arithmetic1 : simulink/Logic and Bit Operations/Shift Arithmetic  SystemSampleTime=-1  nBitShiftRight=7  nBinPtShiftRight=0
  Shift Arithmetic2 : simulink/Logic and Bit Operations/Shift Arithmetic  SystemSampleTime=-1  nBitShiftRight=7  nBinPtShiftRight=0
  Shift Arithmetic3 : simulink/Logic and Bit Operations/Shift Arithmetic  SystemSampleTime=-1  nBitShiftRight=-16  nBinPtShiftRight=0
  Shift Arithmetic4 : simulink/Logic and Bit Operations/Shift Arithmetic  SystemSampleTime=-1  nBitShiftRight=-8  nBinPtShiftRight=0
  Sign : Display
      settings: Format=binary (Stored Integer)
  Subsystem : Subsystem
  Sum : Sum  Inputs=|++
  Sum1 : Sum  Inputs=|+++|
  Sum2 : Sum  Inputs=|+-
  Sum3 : Sum  Inputs=|++
  Out1 : Outport
  wires:
  In4/1 -> Data Type Conversion4/1
  In3/1 -> Data Type Conversion3/1
  Product/1 -> Out1/1
  In1/1 -> Data Type Conversion/1
  Math Function/1 -> Product/1
  Data Type Conversion7/1 -> Math Function/2
  Constant7/1 -> Math Function/1
  Subsystem/1(Out1) -> Product/2
  Data Type Conversion5/1 -> Sum3/2
  Constant5/1 -> Data Type Conversion5/1
  Sum3/1 -> Subsystem/2(In2)
  Sum2/1 -> Subsystem/1(In1)
  Constant4/1 -> Sum2/2
  Sum1/1 -> Sum3/1, Mantissa/1
  Data Type Conversion4/1 -> Sum1/3
  Shift Arithmetic4/1 -> Sum1/2
  Data Type Conversion3/1 -> Shift Arithmetic4/1
  Shift Arithmetic3/1 -> Sum1/1
  Data Type Conversion2/1 -> Bitwise Operator3/1
  Bitwise Operator3/1 -> Shift Arithmetic3/1
  Shift Arithmetic2/1 -> Data Type Conversion7/1, Sign/1
  Bitwise Operator2/1 -> Shift Arithmetic2/1
  Sum/1 -> Sum2/1, Exponent/1
  Shift Arithmetic1/1 -> Sum/2
  Bitwise Operator1/1 -> Shift Arithmetic1/1
  Shift Arithmetic/1 -> Sum/1, Display4/1
  Data Type Conversion1/1 -> Bitwise Operator1/1
  In2/1 -> Data Type Conversion1/1, Data Type Conversion2/1
  Data Type Conversion/1 -> Bitwise Operator2/1, Bitwise Operator/1
  Bitwise Operator/1 -> Shift Arithmetic/1, Display3/1
